simulink model "Lab4a"  (R2023b)
settings: Solver=VariableStepAuto  StartTime=0.0  StopTime=100000.0  RelTol=1e-3
values from neighbouring files (symbols this model uses):
  p12 = 0.3    [Lab4_driver.m]
  p13 = 0.4    [Lab4_driver.m]
  p21 = 0.4    [Lab4_driver.m]
  p33 = 0.2    [Lab4_driver.m]
undefined symbols (not defined in the file or in its folder): control1, control2, control3, m, n
libraries: simulink x2
settings Model: PauseTimes=2  Creator=alberto  LastModifiedBy=alberto

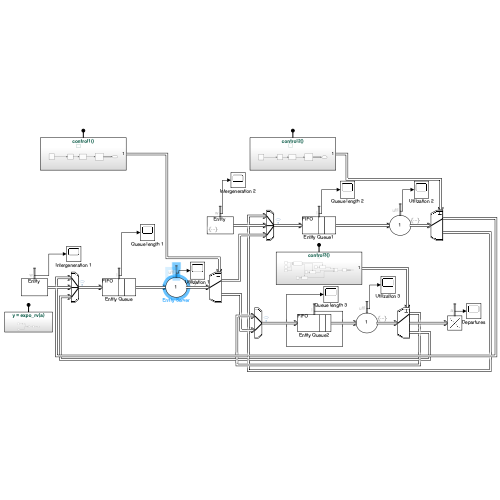
[thumbnail: Simulink's stored preview of the top-level diagram]
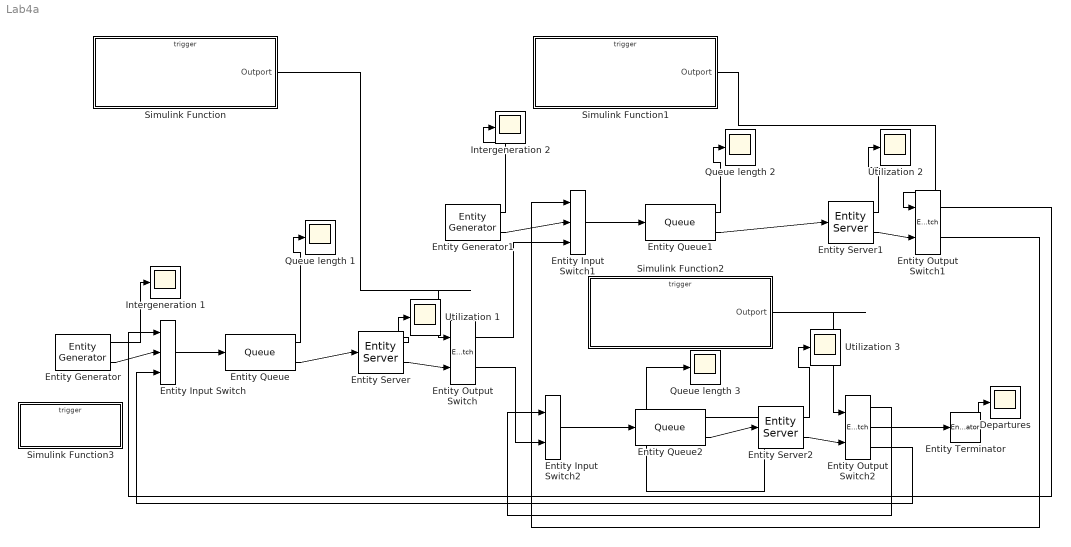
== system Lab4a ==
  Departures : Scope
  Entity Input Switch : EntityInputSwitch  InputPortMessageModes=m,m,m  OutputPortMessageModes=m  NumberInputPorts=3
      settings: InputPortMap=u1,u2,u3
  Entity Input Switch1 : EntityInputSwitch  InputPortMessageModes=m,m,m  OutputPortMessageModes=m  NumberInputPorts=3
      settings: InputPortMap=u1,u2,u3
  Entity Input Switch2 : EntityInputSwitch  InputPortMessageModes=m,m  OutputPortMessageModes=m
  Entity Output Switch : EntityOutputSwitch  InputPortMessageModes=m,m  OutputPortMessageModes=m,m  SwitchingCriterion=From control port  SwitchAttributeName=Attribute1
      settings: InputPortMap=u0,u1
  Entity Output Switch1 : EntityOutputSwitch  InputPortMessageModes=m,m  OutputPortMessageModes=m,m  SwitchingCriterion=From control port  SwitchAttributeName=Attribute1
      settings: InputPortMap=u0,u1
  Entity Output Switch2 : EntityOutputSwitch  InputPortMessageModes=m,m  OutputPortMessageModes=m,m,m  NumberOutputPorts=3  SwitchingCriterion=From control port  SwitchAttributeName=Attribute1
      settings: InputPortMap=u0,u1  OutputPortMap=o0,o1,o2
  Entity Generator : EntityGenerator  OutputPortMessageModes=n,m  TimeSource=MATLAB action  IntergenerationTimeAction=dt = expo_rv(gamma1);  GenerateEntityAtSimulationStart=off  AverageIntergenerationTime=on  EntityType=Structured  EntityTypeName=Entity
      settings: OutputPortMap=o2,o3
  Entity Generator1 : EntityGenerator  OutputPortMessageModes=n,m  TimeSource=MATLAB action  IntergenerationTimeAction=dt = expo_rv(gamma2);  GenerateEntityAtSimulationStart=off  GenerateAction=entity.Attribute1 = 2;  AverageIntergenerationTime=on  EntityType=Structured  EntityTypeName=Entity
      settings: OutputPortMap=o2,o3
  Entity Queue : Queue  InputPortMessageModes=m  OutputPortMessageModes=n,m  Capacity=Inf  AverageQueueLength=on
      settings: OutputPortMap=o3,o5
  Entity Queue1 : Queue  InputPortMessageModes=m  OutputPortMessageModes=n,m  Capacity=Inf  AverageQueueLength=on
      settings: OutputPortMap=o3,o5
  Entity Queue2 : Queue  InputPortMessageModes=m  OutputPortMessageModes=n,m  Capacity=Inf  AverageQueueLength=on
      settings: OutputPortMap=o3,o5
  Entity Server : EntityServer  InputPortMessageModes=m  OutputPortMessageModes=n,m  Capacity=1  ServiceTimeSource=MATLAB action  ServiceTimeAction=dt = expo_rv(mu1);  ExitAction=control1()  Utilization=on
      settings: OutputPortMap=o5,o9
  Entity Server1 : EntityServer  InputPortMessageModes=m  OutputPortMessageModes=n,m  Capacity=1  ServiceTimeSource=MATLAB action  ServiceTimeAction=dt = expo_rv(mu2);  ExitAction=control2()  Utilization=on
      settings: OutputPortMap=o5,o9
  Entity Server2 : EntityServer  InputPortMessageModes=m  OutputPortMessageModes=n,m  Capacity=1  ServiceTimeSource=MATLAB action  ServiceTimeAction=dt = expo_rv(mu3);  ExitAction=control3()  Utilization=on
      settings: OutputPortMap=o5,o9
  Entity Terminator : EntityTerminator  InputPortMessageModes=m  NumberEntitiesArrived=on
      settings: OutputPortMap=o0
  Intergeneration 1 : Scope
  Intergeneration 2 : Scope
  Queue length 1 : Scope
  Queue length 2 : Scope
  Queue length 3 : Scope
  Simulink Function : Subsystem  TreatAsAtomicUnit=on
  Simulink Function1 : Subsystem  TreatAsAtomicUnit=on
  Simulink Function2 : Subsystem  TreatAsAtomicUnit=on
  Simulink Function3 : Subsystem  TreatAsAtomicUnit=on
  Utilization 1 : Scope
  Utilization 2 : Scope
  Utilization 3 : Scope
  wires:
  Entity Generator/2 -> Entity Input Switch/2
  Entity Queue/2 -> Entity Server/1
  Entity Server/2 -> Entity Output Switch/2
  Entity Generator1/2 -> Entity Input Switch1/2
  Entity Queue1/2 -> Entity Server1/1
  Entity Output Switch/1 -> Entity Input Switch1/3
  Entity Server1/2 -> Entity Output Switch1/2
  Entity Output Switch1/1 -> Entity Input Switch/1
  Entity Output Switch/2 -> Entity Input Switch2/2
  Entity Queue2/2 -> Entity Server2/1
  Entity Server2/2 -> Entity Output Switch2/2
  Entity Output Switch2/1 -> Entity Input Switch2/1
  Entity Output Switch2/3 -> Entity Input Switch/3
  Entity Output Switch2/2 -> Entity Terminator/1
  Simulink Function/1(Outport) -> Entity Output Switch/1
  Simulink Function1/1(Outport) -> Entity Output Switch1/1
  Simulink Function2/1(Outport) -> Entity Output Switch2/1
  Entity Server/1 -> Utilization 1/1
  Entity Server1/1 -> Utilization 2/1
  Entity Server2/1 -> Utilization 3/1
  Entity Terminator/1 -> Departures/1
  Entity Generator/1 -> Intergeneration 1/1
  Entity Generator1/1 -> Intergeneration 2/1
  Entity Input Switch1/1 -> Entity Queue1/1
  Entity Output Switch1/2 -> Entity Input Switch1/1
  Entity Input Switch/1 -> Entity Queue/1
  Entity Input Switch2/1 -> Entity Queue2/1
  Entity Queue/1 -> Queue length 1/1
  Entity Queue2/1 -> Queue length 3/1
  Entity Queue1/1 -> Queue length 2/1

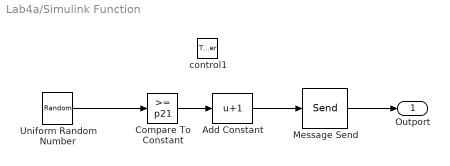
== system Lab4a/Simulink Function ==
  control1 : TriggerPort  TriggerType=function-call  IsSimulinkFunction=on  FunctionName=control1  FunctionVisibility=scoped  VariantControl=(inherit)
  Add Constant : Bias  Bias=1  SaturateOnIntegerOverflow=off
  Compare To Constant : simulink/Logic and Bit Operations/Compare To Constant  relop=>=  const=p21  OutDataTypeStr=uint8
  Message Send : Send  OutputPortMessageModes=m
  Uniform Random Number : UniformRandomNumber  Minimum=0  Seed=randi(3750)
  Outport : Outport
  wires:
  Compare To Constant/1 -> Add Constant/1
  Uniform Random Number/1 -> Compare To Constant/1
  Add Constant/1 -> Message Send/1
  Message Send/1 -> Outport/1

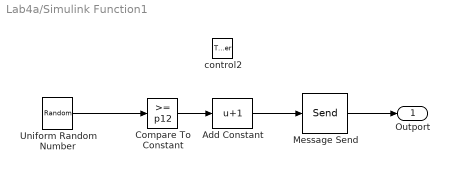
== system Lab4a/Simulink Function1 ==
  control2 : TriggerPort  TriggerType=function-call  IsSimulinkFunction=on  FunctionName=control2  FunctionVisibility=scoped  VariantControl=(inherit)
  Add Constant : Bias  Bias=1  SaturateOnIntegerOverflow=off
  Compare To Constant : simulink/Logic and Bit Operations/Compare To Constant  relop=>=  const=p12  OutDataTypeStr=uint8
  Message Send : Send  OutputPortMessageModes=m
  Uniform Random Number : UniformRandomNumber  Minimum=0  Seed=randi(3750)
  Outport : Outport
  wires:
  Compare To Constant/1 -> Add Constant/1
  Uniform Random Number/1 -> Compare To Constant/1
  Add Constant/1 -> Message Send/1
  Message Send/1 -> Outport/1

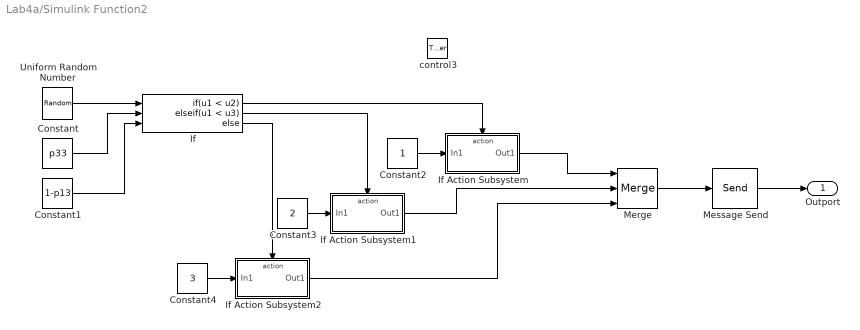
== system Lab4a/Simulink Function2 ==
  control3 : TriggerPort  TriggerType=function-call  IsSimulinkFunction=on  FunctionName=control3  FunctionVisibility=scoped  VariantControl=(inherit)
  Constant : Constant  Value=p33  SampleTime=-1
  Constant1 : Constant  Value=1-p13  SampleTime=-1
  Constant2 : Constant  SampleTime=-1
  Constant3 : Constant  Value=2  SampleTime=-1
  Constant4 : Constant  Value=3  SampleTime=-1
  If : If  NumInputs=3  IfExpression=u1 < u2  ElseIfExpressions=u1 < u3
  If Action Subsystem : Subsystem  TreatAsAtomicUnit=on
  If Action Subsystem1 : Subsystem  TreatAsAtomicUnit=on
  If Action Subsystem2 : Subsystem  TreatAsAtomicUnit=on
  Merge : Merge  Inputs=3
  Message Send : Send  OutputPortMessageModes=m
  Uniform Random Number : UniformRandomNumber  Minimum=0  Seed=randi(3750)
  Outport : Outport
  wires:
  Uniform Random Number/1 -> If/1
  Merge/1 -> Message Send/1
  Message Send/1 -> Outport/1
  Constant/1 -> If/2
  Constant1/1 -> If/3
  If Action Subsystem/1(Out1) -> Merge/1
  If/1 -> If Action Subsystem/Action
  If/2 -> If Action Subsystem1/Action
  If/3 -> If Action Subsystem2/Action
  If Action Subsystem1/1(Out1) -> Merge/2
  If Action Subsystem2/1(Out1) -> Merge/3
  Constant2/1 -> If Action Subsystem/1(In1)
  Constant3/1 -> If Action Subsystem1/1(In1)
  Constant4/1 -> If Action Subsystem2/1(In1)

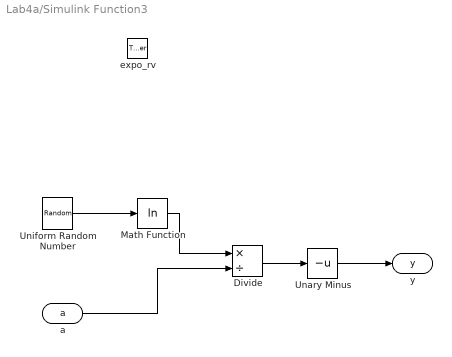
== system Lab4a/Simulink Function3 ==
  expo_rv : TriggerPort  TriggerType=function-call  IsSimulinkFunction=on  FunctionName=expo_rv  FunctionVisibility=scoped  VariantControl=(inherit)
  Divide : Product  Inputs=*/
  Math Function : Math  Operator=log
  Unary Minus : UnaryMinus
  Uniform Random Number : UniformRandomNumber  Minimum=0  VectorParams1D=off
  a : ArgIn  DisableCoverage=on  ArgumentName=a
  y : ArgOut  DisableCoverage=on  ArgumentName=y
  wires:
  a/1 -> Divide/2
  Uniform Random Number/1 -> Math Function/1
  Math Function/1 -> Divide/1
  Divide/1 -> Unary Minus/1
  Unary Minus/1 -> y/1

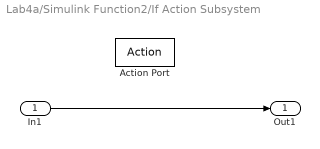
== system Lab4a/Simulink Function2/If Action Subsystem ==
  In1 : Inport
  Action Port : ActionPort  ActionPortLabel=if(u1 < u2)
  Out1 : Outport
  wires:
  In1/1 -> Out1/1

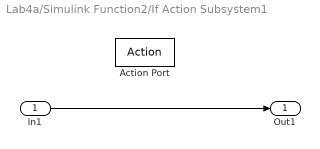
== system Lab4a/Simulink Function2/If Action Subsystem1 ==
  In1 : Inport
  Action Port : ActionPort  ActionPortLabel=elseif(u1 < u3)
  Out1 : Outport
  wires:
  In1/1 -> Out1/1

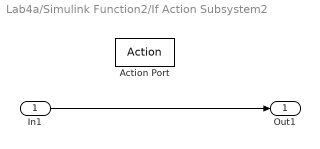
== system Lab4a/Simulink Function2/If Action Subsystem2 ==
  In1 : Inport
  Action Port : ActionPort  ActionPortLabel=else
  Out1 : Outport
  wires:
  In1/1 -> Out1/1
